simulink model "model1_副本"  (R2023b)
settings: Solver=VariableStepAuto  StartTime=0.0  StopTime=10.0  RelTol=1e-3
undefined symbols (not defined in the file): a558, b523fd510067, DiscIntNeverNeededParam, e0d6, magnitude, Newton, Raphson
libraries: simulink x87, slpidlib x16
(part 1 of 3)
settings Model: Creator=OSCAR4  LastModifiedBy=OSCAR4

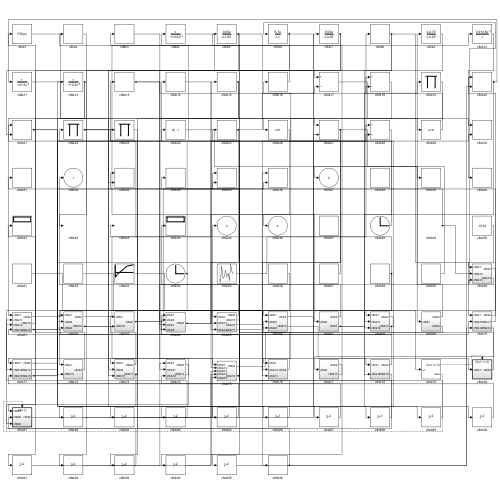
[thumbnail: Simulink's stored preview of the top-level diagram]
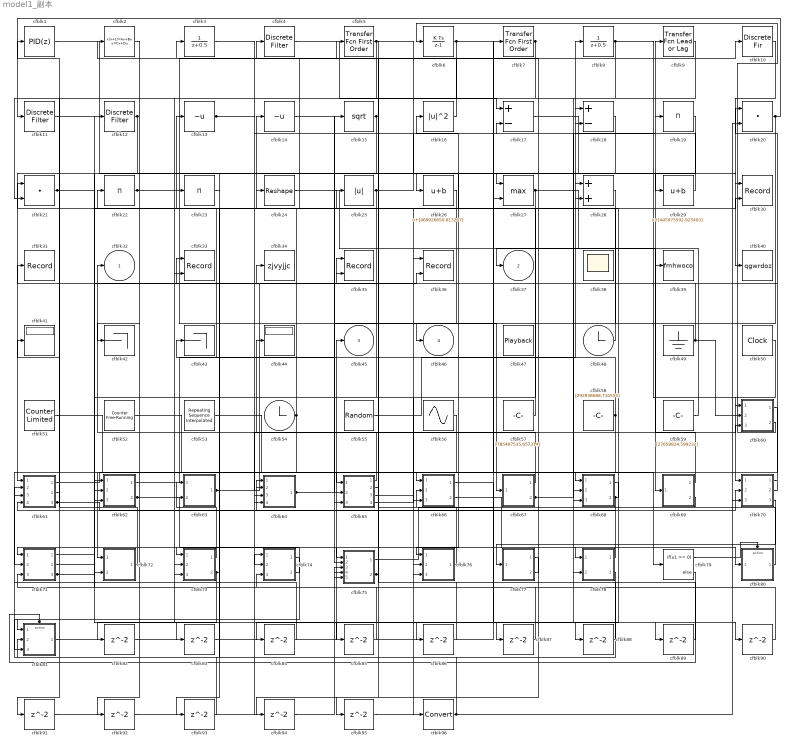
== system model1_副本 ==
  cfblk1 : slpidlib/PID Controller  Controller=PID  Form=Parallel  TimeDomain=Discrete-time  UseExternalTs=off  SampleTime=1  IntegratorMethod=Forward Euler  FilterMethod=Forward Euler  ControllerParametersSource=internal  P=1  I=1  UseKiTs=off  D=0  N=100  UseFilter=on  TunerSelectOption=Transfer Function Based (PID Tuner App)  InitialConditionSource=internal  InitialConditionForIntegrator=0  InitialConditionForFilter=0  DifferentiatorICPrevScaledInput=0  ExternalReset=none  TrackingMode=off  Kt=1  LimitOutput=off  SatLimitsSource=internal  UpperSaturationLimit=inf  LowerSaturationLimit=-inf  LinearizeAsGain=off  AntiWindupMode=none  Kb=1  LimitIntegrator=off  UpperIntegratorSaturationLimit=inf  LowerIntegratorSaturationLimit=-inf  POutMin=[]  POutMax=[]  IOutMin=[]  IOutMax=[]  DOutMin=[]  DOutMax=[]  NOutMin=[]  NOutMax=[]  SumOutMin=[]  SumOutMax=[]  SaturationOutMin=[]  SaturationOutMax=[]  PParamMin=[]  PParamMax=[]  IParamMin=[]  IParamMax=[]  DParamMin=[]  DParamMax=[]  NParamMin=[]  NParamMax=[]  KbParamMin=[]  KbParamMax=[]  KtParamMin=[]  KtParamMax=[]  KbOutMin=[]  KbOutMax=[]  KtOutMin=[]  KtOutMax=[]  IntegratorOutMin=[]  IntegratorOutMax=[]  FilterOutMin=[]  FilterOutMax=[]  SumI1OutMin=[]  SumI1OutMax=[]  SumI2OutMin=[]  SumI2OutMax=[]  SumI3OutMin=[]  SumI3OutMax=[]  SumI4OutMin=[]  SumI4OutMax=[]  SumDOutMin=[]  SumDOutMax=[]  DifferentiatorOutMin=[]  DifferentiatorOutMax=[]  FilterDiffOutCoefMin=[]  FilterDiffOutCoefMax=[]  ReciprocalOutMin=[]  ReciprocalOutMax=[]  SumDenOutMin=[]  SumDenOutMax=[]  SumNumOutMin=[]  SumNumOutMax=[]  DivideOutMin=[]  DivideOutMax=[]  UdiffTsProdOutMin=[]  UdiffTsProdOutMax=[]  NTsProdOutMin=[]  NTsProdOutMax=[]  UintegralTsProdOutMin=[]  UintegralTsProdOutMax=[]  UngainTsProdOutMin=[]  UngainTsProdOutMax=[]  ClampingZeroOutDataTypeStr=Inherit: Inherit via back propagation  ClampingZeroOutMin=[]  ClampingZeroOutMax=[]  FilterDenConstantOutDataTypeStr=Inherit: Inherit via back propagation  FilterDenConstantOutMin=[]  FilterDenConstantOutMax=[]  PCopyOutDataTypeStr=Inherit: Inherit via back propagation  PCopyOutMin=[]  PCopyOutMax=[]  NCopyOutDataTypeStr=Inherit: Inherit via back propagation  NCopyOutMin=[]  NCopyOutMax=[]  IntegratorContinuousStateAttributes=''  IntegratorStateMustResolveToSignalObject=off  IntegratorRTWStateStorageClass=Auto  FilterContinuousStateAttributes=''  FilterStateMustResolveToSignalObject=off  FilterRTWStateStorageClass=Auto  ParallelPVariant=InternalParameters  IdealPVariant=Disabled  IVariant=InternalParameters  DVariant=InternalParameters  IntegratorVariant=Discrete  SatVariant=Disabled  AWVariant=Passthrough  PCopyVariant=Disabled  TRVariant=Disabled  FdbkBlocksVariant=Forward  IdealPFdbkVariant=Disabled  SatFdbkVariant=Disabled  DerivativeFilterVariant=ForwardEulerFilter  NVariant=InternalParameters  NCopyVariant=Disabled  FilterICVariant=InternalICsFilter  IntegratorICVariant=InternalICs  ExternalResetVariant=Disabled  TRSumVariant=Passthrough  SumFdbkVariant=Disabled  SumVariant=Sum_PID  TsampFilterVariant=InternalTs  TsampNgainVariant=Passthrough  TsampIntegralVariant=Disabled_SignalSpec  ExternalSaturationOutDataTypeStr=Inherit: Same as second input
      settings: LibrarySourceBlock=simulink/Discrete/Discrete PID Controller
  cfblk10 : DiscreteFir  SampleTime=1
  cfblk11 : DiscreteFilter  SampleTime=1
  cfblk12 : DiscreteFilter  SampleTime=1
  cfblk13 : UnaryMinus
  cfblk14 : UnaryMinus
  cfblk15 : Sqrt
  cfblk16 : Math  Operator=magnitude^2
  cfblk17 : Sum  Inputs=+-
  cfblk18 : Sum  Inputs=+-
  cfblk19 : Product  Inputs=*
  cfblk2 : DiscreteStateSpace
  cfblk20 : DotProduct  OutDataTypeStr=Inherit: Inherit via internal rule
  cfblk21 : DotProduct  OutDataTypeStr=Inherit: Inherit via internal rule
  cfblk22 : Product  Inputs=*
  cfblk23 : Product  Inputs=*
  cfblk24 : Reshape
  cfblk25 : Abs  SaturateOnIntegerOverflow=off
  cfblk26 : Bias  Bias=[469926650.613267]  SaturateOnIntegerOverflow=off
  cfblk27 : MinMax  Function=max  Inputs=2
  cfblk28 : Sum
  cfblk29 : Bias  Bias=[445975592.923403]  SaturateOnIntegerOverflow=off
  cfblk3 : DiscreteTransferFcn  SampleTime=1
  cfblk30 : Record  FileSettingsInternal="{\"entries\":[{\"content\":{\"excelSettings\":{\"content\":{},\"type\":\"Streamout.ExcelSettings\"}},\"type\":\"Streamout.FileSettingStorage\",\"uuid\":\"\"}],\"packageUris\":[\"http:\\/\\/schema.mathworks.com\\/mf0\\/streamout_blocks\\/R2020a\"],\"version\":\"1.0\"}"  Layout=[1 1]  SignalsInternal="{\"entries\":[{\"content\":{\"signals\":[{\"content\":{\"blockPath\":[],\"dimensions\":[1],\"domain\":\"\",\"lineColor\":\"#a2142f\",\"plots\":[1],\"port\":1,\"sid\":[\"\"],\"signalID\":864,\"signalName\":\"cfblk17\"},\"type\":\"RecordBlkView.Signal\",\"uuid\":\"\"},{\"content\":{\"blockPath\":[],\"dimensions\":[1],\"domain\":\"\",\"lineColor\":\"#139fff\",\"plots\":[1],\"port\":2,\"sid\":[\"\"],\"signalID\":868,\"signalName\":\"cfblk65:3\"},\"type\":\"RecordBlkView.Signal\",\"uuid\":\"\"}]},\"type\":\"RecordBlkView.InputSignals\",\"uuid\":\"\"}],\"packageUris\":[\"http:\\/\\/schema.mathworks.com\\/mf0\\/streamout_blocks\\/R2020a\"],\"version\":\"1.0\"}"  VisualizationBindings="{\"xyplotplugin\":{\"info\":[{\"series\":[{\"bindingParametersList\":[{\"parameter\":\"X-Axis\",\"signalID\":864,\"signalName\":\"cfblk17\"},{\"parameter\":\"Y-Axis\",\"signalID\":868,\"signalName\":\"cfblk65:3\"}],\"seriesID\":27169}],\"subplotID\":1}]}}"  CompatibilityTag=XY
  cfblk31 : Record  FileSettingsInternal="{\"entries\":[{\"content\":{\"excelSettings\":{\"content\":{},\"type\":\"Streamout.ExcelSettings\"}},\"type\":\"Streamout.FileSettingStorage\",\"uuid\":\"\"}],\"packageUris\":[\"http:\\/\\/schema.mathworks.com\\/mf0\\/streamout_blocks\\/R2020a\"],\"version\":\"1.0\"}"  SignalsInternal="{\"entries\":[{\"content\":{\"signals\":[{\"content\":{\"blockPath\":[],\"dimensions\":[1],\"domain\":\"\",\"lineColor\":\"#ff6929\",\"plots\":[1],\"port\":1,\"sid\":[\"\"],\"signalID\":848,\"signalName\":\"cfblk75:2\"},\"type\":\"RecordBlkView.Signal\",\"uuid\":\"\"}]},\"type\":\"RecordBlkView.InputSignals\",\"uuid\":\"\"}],\"packageUris\":[\"http:\\/\\/schema.mathworks.com\\/mf0\\/streamout_blocks\\/R2020a\"],\"version\":\"1.0\"}"  VisualizationBindings="{\"sparklinesplugin\":{\"info\":[{\"bindingParametersList\":[],\"subplotID\":1}]}}"
  cfblk33 : Record  FileSettingsInternal="{\"entries\":[{\"content\":{\"excelSettings\":{\"content\":{},\"type\":\"Streamout.ExcelSettings\"}},\"type\":\"Streamout.FileSettingStorage\",\"uuid\":\"\"}],\"packageUris\":[\"http:\\/\\/schema.mathworks.com\\/mf0\\/streamout_blocks\\/R2020a\"],\"version\":\"1.0\"}"  Layout=[1 1]  SignalsInternal="{\"entries\":[{\"content\":{\"signals\":[{\"content\":{\"blockPath\":[],\"dimensions\":[1],\"domain\":\"\",\"lineColor\":\"#a2142f\",\"plots\":[1],\"port\":1,\"sid\":[\"\"],\"signalID\":872,\"signalName\":\"cfblk75:2\"},\"type\":\"RecordBlkView.Signal\",\"uuid\":\"\"},{\"content\":{\"blockPath\":[],\"dimensions\":[1],\"domain\":\"\",\"lineColor\":\"#139fff\",\"plots\":[1],\"port\":2,\"sid\":[\"\"],\"signalID\":876,\"signalName\":\"cfblk8\"},\"type\":\"RecordBlkView.Signal\",\"uuid\":\"\"}]},\"type\":\"RecordBlkView.InputSignals\",\"uuid\":\"\"}],\"packageUris\":[\"http:\\/\\/schema.mathworks.com\\/mf0\\/streamout_blocks\\/R2020a\"],\"version\":\"1.0\"}"  VisualizationBindings="{\"xyplotplugin\":{\"info\":[{\"series\":[{\"bindingParametersList\":[{\"parameter\":\"X-Axis\",\"signalID\":872,\"signalName\":\"cfblk75:2\"},{\"parameter\":\"Y-Axis\",\"signalID\":876,\"signalName\":\"cfblk8\"}],\"seriesID\":2036}],\"subplotID\":1}]}}"  CompatibilityTag=XY
  cfblk34 : ToWorkspace  VariableName=zjvyjjc  SaveFormat=Timeseries  SampleTime=-1
  cfblk35 : Record  FileSettingsInternal="{\"entries\":[{\"content\":{\"excelSettings\":{\"content\":{},\"type\":\"Streamout.ExcelSettings\"}},\"type\":\"Streamout.FileSettingStorage\",\"uuid\":\"\"}],\"packageUris\":[\"http:\\/\\/schema.mathworks.com\\/mf0\\/streamout_blocks\\/R2020a\"],\"version\":\"1.0\"}"  Layout=[1 1]  SignalsInternal="{\"entries\":[{\"content\":{\"signals\":[{\"content\":{\"blockPath\":[],\"dimensions\":[1],\"domain\":\"\",\"lineColor\":\"#139fff\",\"plots\":[1],\"port\":2,\"sid\":[\"\"],\"signalID\":880,\"signalName\":\"cfblk63\"},\"type\":\"RecordBlkView.Signal\",\"uuid\":\"\"},{\"content\":{\"blockPath\":[],\"dimensions\":[1],\"domain\":\"\",\"lineColor\":\"#a2142f\",\"plots\":[1],\"port\":1,\"sid\":[\"\"],\"signalID\":896,\"signalName\":\"cfblk49\"},\"type\":\"RecordBlkView.Signal\",\"uuid\":\"\"}]},\"type\":\"RecordBlkView.InputSignals\",\"uuid\":\"\"}],\"packageUris\":[\"http:\\/\\/schema.mathworks.com\\/mf0\\/streamout_blocks\\/R2020a\"],\"version\":\"1.0\"}"  VisualizationBindings="{\"xyplotplugin\":{\"info\":[{\"series\":[{\"bindingParametersList\":[{\"parameter\":\"X-Axis\",\"signalID\":896,\"signalName\":\"cfblk49\"},{\"parameter\":\"Y-Axis\",\"signalID\":880,\"signalName\":\"cfblk63\"}],\"seriesID\":60971}],\"subplotID\":1}]}}"  CompatibilityTag=XY
  cfblk36 : Record  FileSettingsInternal="{\"entries\":[{\"content\":{\"excelSettings\":{\"content\":{},\"type\":\"Streamout.ExcelSettings\"}},\"type\":\"Streamout.FileSettingStorage\",\"uuid\":\"\"}],\"packageUris\":[\"http:\\/\\/schema.mathworks.com\\/mf0\\/streamout_blocks\\/R2020a\"],\"version\":\"1.0\"}"  Layout=[1 1]  SignalsInternal="{\"entries\":[{\"content\":{\"signals\":[{\"content\":{\"blockPath\":[],\"dimensions\":[1,1],\"domain\":\"\",\"lineColor\":\"#a2142f\",\"plots\":[1],\"port\":1,\"sid\":[\"\"],\"signalID\":884,\"signalName\":\"cfblk65:4\"},\"type\":\"RecordBlkView.Signal\",\"uuid\":\"\"},{\"content\":{\"blockPath\":[],\"dimensions\":[1,1],\"domain\":\"\",\"lineColor\":\"#139fff\",\"plots\":[1],\"port\":2,\"sid\":[\"\"],\"signalID\":888,\"signalName\":\"cfblk71:3\"},\"type\":\"RecordBlkView.Signal\",\"uuid\":\"\"}]},\"type\":\"RecordBlkView.InputSignals\",\"uuid\":\"\"}],\"packageUris\":[\"http:\\/\\/schema.mathworks.com\\/mf0\\/streamout_blocks\\/R2020a\"],\"version\":\"1.0\"}"  VisualizationBindings="{\"xyplotplugin\":{\"info\":[{\"series\":[{\"bindingParametersList\":[{\"parameter\":\"X-Axis\",\"signalID\":884,\"signalName\":\"cfblk65:4\"},{\"parameter\":\"Y-Axis\",\"signalID\":888,\"signalName\":\"cfblk71:3\"}],\"seriesID\":23987}],\"subplotID\":1}]}}"  CompatibilityTag=XY
  cfblk38 : Scope
      settings: Floating=on
  cfblk39 : ToWorkspace  VariableName=fmhwoco  SaveFormat=Timeseries  SampleTime=-1
  cfblk4 : DiscreteFilter  SampleTime=1
  cfblk40 : ToWorkspace  VariableName=qgwrdoz  SaveFormat=Timeseries  SampleTime=-1
  cfblk41 : Display
  cfblk42 : Terminator
  cfblk43 : Terminator
  cfblk44 : Display
  cfblk47 : Playback  NumPorts=0  PartName=36defed5-e0d6-41a1-a558-b523fd510067
  cfblk48 : Clock
  cfblk49 : Ground
  cfblk5 : simulink/Discrete/Transfer Fcn First Order  PoleZ=0.95  ICPrevOutput=0.0  DoSatur=off
  cfblk50 : DigitalClock
  cfblk51 : simulink/Sources/Counter Limited  uplimit=[223.000000]  tsamp=-1
  cfblk52 : simulink/Sources/Counter Free-Running  NumBits=[22.000000]  tsamp=-1
  cfblk53 : simulink/Sources/Repeating Sequence Interpolated  OutValues=[-505600590.852767, -222429001.362350, 434169832.894922, 629003669.042864, 798997869.181004]  TimeValues=[0 0.1 0.5 0.6 1].'  LookUpMeth=Use Input Nearest  tsamp=0.01  OutMin=[]  OutMax=[]  OutDataTypeStr=double  OutputDataTypeScalingMode=double  OutDataType=fixdt(0,8)  OutScaling=2^-10
  cfblk54 : Clock
  cfblk55 : UniformRandomNumber  Minimum=[-9244758245.197369]  Maximum=[3053319660.851500]  Seed=[9943217.000000]  SampleTime=0.1
  cfblk56 : Sin  Amplitude=[-790585520.472188]  Bias=[947156710.319980]  SampleTime=0
  cfblk57 : Constant  Value=[785497535.657314]  SampleTime=1
  cfblk58 : Constant  Value=[292938688.710555]  SampleTime=1
  cfblk59 : Constant  Value=[27658824.599232]  SampleTime=1
  cfblk6 : DiscreteIntegrator  ICPrevOutput=DiscIntNeverNeededParam  ICPrevScaledInput=DiscIntNeverNeededParam
  cfblk60 : Subsystem
  cfblk61 : Subsystem
  cfblk62 : Subsystem
  cfblk63 : Subsystem
  cfblk64 : Subsystem
  cfblk65 : Subsystem
  cfblk66 : Subsystem
  cfblk67 : Subsystem
  cfblk68 : Subsystem
  cfblk69 : Subsystem
  cfblk7 : simulink/Discrete/Transfer Fcn First Order  PoleZ=0.95  ICPrevOutput=0.0  DoSatur=off
  cfblk70 : Subsystem
  cfblk71 : Subsystem
  cfblk72 : Subsystem
  cfblk73 : Subsystem
  cfblk74 : Subsystem
  cfblk75 : Subsystem
  cfblk76 : Subsystem
  cfblk77 : Subsystem
  cfblk78 : Subsystem
  cfblk79 : If  IfExpression=u1 >= 0  SampleTime=1
  cfblk8 : DiscreteTransferFcn  SampleTime=1
  cfblk80 : Subsystem  TreatAsAtomicUnit=on
  cfblk81 : Subsystem  TreatAsAtomicUnit=on
  cfblk{82..95} (14 alike) : Delay  SampleTime=1
  cfblk9 : simulink/Discrete/Transfer Fcn Lead or Lag  PoleZ=0.95  ZeroZ=0.75  ICPrevOutput=0.0  ICPrevInput=0.0  DoSatur=off
  cfblk96 : DataTypeConversion  SaturateOnIntegerOverflow=off  RndMeth=Floor
  cfblk32 : Outport
  cfblk37 : Outport  Port=2
  cfblk45 : Outport  Port=3
  cfblk46 : Outport  Port=4
  wires:
  cfblk81/1(cfblk2) -> cfblk45/1
  cfblk52/1 -> cfblk96/1
  cfblk1/1 -> cfblk26/1
  cfblk49/1 -> cfblk35/1, cfblk60/2(cfblk12)
  cfblk61/1(cfblk2) -> cfblk65/1(cfblk1)
  cfblk60/1(cfblk2) -> cfblk65/2(cfblk13)
  cfblk54/1 -> cfblk14/1, cfblk64/3(cfblk7)
  cfblk22/1 -> cfblk10/1, cfblk67/1(cfblk1), cfblk90/1
  cfblk62/1(cfblk2) -> cfblk15/1
  cfblk26/1 -> cfblk46/1
  cfblk64/1(cfblk2) -> cfblk66/1(cfblk1), cfblk28/1
  cfblk59/1 -> cfblk37/1
  cfblk16/1 -> cfblk2/1
  cfblk28/1 -> cfblk65/3(cfblk14)
  cfblk63/1(cfblk2) -> cfblk35/2, cfblk60/3(cfblk13)
  cfblk29/1 -> cfblk8/1
  cfblk57/1 -> cfblk4/1
  cfblk69/1(cfblk2) -> cfblk9/1
  cfblk75/1(cfblk2) -> cfblk7/1
  cfblk24/1 -> cfblk69/1(cfblk1)
  cfblk65/1(cfblk2) -> cfblk32/1
  cfblk15/1 -> cfblk61/1(cfblk1), cfblk64/4(cfblk8)
  cfblk60/2(cfblk14) -> cfblk6/1
  cfblk50/1 -> cfblk70/1(cfblk1)
  cfblk51/1 -> cfblk79/1
  cfblk62/2(cfblk10) -> cfblk78/1(cfblk1), cfblk63/2(cfblk16)
  cfblk12/1 -> cfblk81/1(cfblk1), cfblk62/3(cfblk9)
  cfblk69/2(cfblk8) -> cfblk66/2(cfblk8)
  cfblk5/1 -> cfblk29/1, cfblk73/3(cfblk10), cfblk95/1
  cfblk14/1 -> cfblk66/3(cfblk9)
  cfblk48/1 -> cfblk16/1
  cfblk10/1 -> cfblk40/1
  cfblk9/1 -> cfblk78/2(cfblk15)
  cfblk6/1 -> cfblk68/1(cfblk1), cfblk91/1
  cfblk13/1 -> cfblk75/1(cfblk1), cfblk18/2
  cfblk20/1 -> cfblk11/1, cfblk68/2(cfblk11)
  cfblk27/1 -> cfblk75/2(cfblk12), cfblk39/1, cfblk76/3(cfblk11)
  cfblk73/1(cfblk2) -> cfblk63/1(cfblk1)
  cfblk8/1 -> cfblk60/1(cfblk1), cfblk21/2, cfblk33/2
  cfblk56/1 -> cfblk72/1(cfblk1)
  cfblk80/1(cfblk2) -> cfblk22/1
  cfblk76/1(cfblk2) -> cfblk25/1
  cfblk3/1 -> cfblk27/1
  cfblk58/1 -> cfblk13/1, cfblk71/2(cfblk10), cfblk68/3(cfblk12)
  cfblk78/1(cfblk2) -> cfblk64/1(cfblk1)
  cfblk78/2(cfblk16) -> cfblk81/2(cfblk8)
  cfblk70/1(cfblk2) -> cfblk20/1
  cfblk4/1 -> cfblk17/1
  cfblk18/1 -> cfblk73/1(cfblk1)
  cfblk11/1 -> cfblk73/2(cfblk9)
  cfblk74/1(cfblk2) -> cfblk81/3(cfblk9)
  cfblk73/2(cfblk11) -> cfblk23/1, cfblk92/1
  cfblk21/1 -> cfblk86/1, cfblk87/1
  cfblk70/2(cfblk13) -> cfblk34/1
  cfblk17/1 -> cfblk30/1
  cfblk7/1 -> cfblk74/2(cfblk11), cfblk82/1
  cfblk2/1 -> cfblk42/1
  cfblk25/1 -> cfblk17/2, cfblk72/2(cfblk10)
  cfblk70/3(cfblk14) -> cfblk77/1(cfblk1)
  cfblk55/1 -> cfblk18/1
  cfblk74/2(cfblk13) -> cfblk71/1(cfblk1)
  cfblk66/2(cfblk10) -> cfblk80/1(cfblk1)
  cfblk19/1 -> cfblk76/1(cfblk1)
  cfblk71/2(cfblk12) -> cfblk12/1
  cfblk75/2(cfblk16) -> cfblk31/1, cfblk33/1
  cfblk53/1 -> cfblk76/2(cfblk10)
  cfblk67/1(cfblk2) -> cfblk44/1
  cfblk77/2(cfblk17) -> cfblk5/1
  cfblk68/2(cfblk13) -> cfblk21/1, cfblk64/2(cfblk6)
  cfblk65/3(cfblk16) -> cfblk30/2
  cfblk61/2(cfblk14) -> cfblk1/1
  cfblk65/4(cfblk17) -> cfblk36/1
  cfblk71/3(cfblk13) -> cfblk24/1, cfblk36/2
  cfblk72/1(cfblk2) -> cfblk41/1
  cfblk61/3(cfblk15) -> cfblk70/2(cfblk11), cfblk28/2
  cfblk67/2(cfblk7) -> cfblk19/1, cfblk89/1
  cfblk79/1 -> cfblk80/Action
  cfblk79/2 -> cfblk81/Action
  cfblk82/1 -> cfblk27/2
  cfblk71/1(cfblk2) -> cfblk83/1
  cfblk83/1 -> cfblk75/3(cfblk13)
  cfblk65/2(cfblk15) -> cfblk84/1
  cfblk84/1 -> cfblk61/3(cfblk12)
  cfblk68/1(cfblk2) -> cfblk85/1
  cfblk85/1 -> cfblk62/2(cfblk8)
  cfblk86/1 -> cfblk3/1
  cfblk87/1 -> cfblk74/3(cfblk12)
  cfblk66/1(cfblk2) -> cfblk88/1
  cfblk88/1 -> cfblk62/1(cfblk1)
  cfblk89/1 -> cfblk61/4(cfblk13)
  cfblk90/1 -> cfblk71/3(cfblk11)
  cfblk91/1 -> cfblk75/5(cfblk15)
  cfblk92/1 -> cfblk74/1(cfblk1)
  cfblk23/1 -> cfblk93/1
  cfblk93/1 -> cfblk61/2(cfblk11)
  cfblk77/1(cfblk2) -> cfblk94/1
  cfblk94/1 -> cfblk75/4(cfblk14)
  cfblk95/1 -> cfblk70/3(cfblk12)
  cfblk96/1 -> cfblk20/2, cfblk43/1

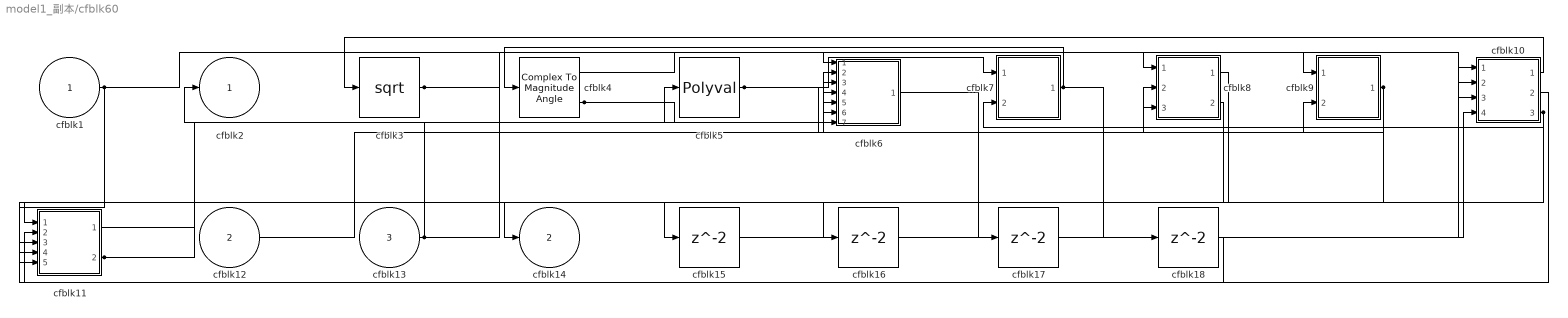
== system model1_副本/cfblk60 ==
  cfblk1 : Inport
  cfblk12 : Inport  Port=2
  cfblk13 : Inport  Port=3
  cfblk10 : Subsystem
  cfblk11 : Subsystem
  cfblk{15..18} (4 alike) : Delay  SampleTime=1
  cfblk3 : Sqrt
  cfblk4 : ComplexToMagnitudeAngle
  cfblk5 : Polyval  Coefs=[ +2.081618890e-019, -1.441693666e-014, +4.719686976e-010, -8.536869453e-006, +1.621573104e-001, -8.087801117e+001 ]
  cfblk6 : Subsystem
  cfblk7 : Subsystem
  cfblk8 : Subsystem
  cfblk9 : Subsystem
  cfblk2 : Outport
  cfblk14 : Outport  Port=2
  wires:
  cfblk5/1 -> cfblk7/1(cfblk1), cfblk9/2(cfblk7)
  cfblk7/1(cfblk2) -> cfblk4/1, cfblk18/1
  cfblk9/1(cfblk2) -> cfblk14/1, cfblk6/6(cfblk16)
  cfblk13/1 -> cfblk2/1, cfblk6/4(cfblk14), cfblk8/3(cfblk15)
  cfblk4/1 -> cfblk6/1(cfblk1)
  cfblk10/1(cfblk2) -> cfblk3/1
  cfblk8/2(cfblk16) -> cfblk11/1(cfblk1)
  cfblk1/1 -> cfblk10/3(cfblk14), cfblk11/3(cfblk9), cfblk9/1(cfblk1)
  cfblk3/1 -> cfblk8/1(cfblk1), cfblk6/5(cfblk15)
  cfblk12/1 -> cfblk8/2(cfblk14)
  cfblk4/2 -> cfblk6/2(cfblk12), cfblk6/7(cfblk17)
  cfblk10/2(cfblk16) -> cfblk11/2(cfblk8)
  cfblk11/2(cfblk12) -> cfblk6/3(cfblk13), cfblk5/1
  cfblk10/3(cfblk17) -> cfblk7/2(cfblk9), cfblk11/5(cfblk11)
  cfblk8/1(cfblk2) -> cfblk15/1
  cfblk15/1 -> cfblk10/1(cfblk1)
  cfblk11/1(cfblk2) -> cfblk16/1
  cfblk16/1 -> cfblk10/4(cfblk15)
  cfblk6/1(cfblk2) -> cfblk17/1
  cfblk17/1 -> cfblk10/2(cfblk13)
  cfblk18/1 -> cfblk11/4(cfblk10)

== system model1_副本/cfblk61 ==
  cfblk1 : Inport
  cfblk11 : Inport  Port=2
  cfblk12 : Inport  Port=3
  cfblk13 : Inport  Port=4
  cfblk10 : Subsystem
  cfblk16 : Delay  SampleTime=1
  cfblk3 : simulink/Discrete/Transfer Fcn First Order  PoleZ=0.95  ICPrevOutput=0.0  DoSatur=off
  cfblk4 : slpidlib/PID Controller (2DOF)  Controller=PID  Form=Parallel  TimeDomain=Discrete-time  UseExternalTs=off  SampleTime=1  IntegratorMethod=Forward Euler  FilterMethod=Forward Euler  ControllerParametersSource=internal  P=1  I=1  UseKiTs=off  D=0  N=100  UseFilter=on  b=1  c=1  TunerSelectOption=Transfer Function Based (PID Tuner App)  InitialConditionSource=internal  InitialConditionForIntegrator=0  InitialConditionForFilter=0  DifferentiatorICPrevScaledInput=0  ExternalReset=none  TrackingMode=off  Kt=1  LimitOutput=off  SatLimitsSource=internal  UpperSaturationLimit=inf  LowerSaturationLimit=-inf  LinearizeAsGain=off  AntiWindupMode=none  Kb=1  LimitIntegrator=off  UpperIntegratorSaturationLimit=inf  LowerIntegratorSaturationLimit=-inf  POutMin=[]  POutMax=[]  IOutMin=[]  IOutMax=[]  DOutMin=[]  DOutMax=[]  NOutMin=[]  NOutMax=[]  bOutMin=[]  bOutMax=[]  cOutMin=[]  cOutMax=[]  SumOutMin=[]  SumOutMax=[]  SaturationOutMin=[]  SaturationOutMax=[]  PParamMin=[]  PParamMax=[]  IParamMin=[]  IParamMax=[]  DParamMin=[]  DParamMax=[]  NParamMin=[]  NParamMax=[]  bParamMin=[]  bParamMax=[]  cParamMin=[]  cParamMax=[]  KbParamMin=[]  KbParamMax=[]  KtParamMin=[]  KtParamMax=[]  KbOutMin=[]  KbOutMax=[]  KtOutMin=[]  KtOutMax=[]  IntegratorOutMin=[]  IntegratorOutMax=[]  FilterOutMin=[]  FilterOutMax=[]  SumI1OutMin=[]  SumI1OutMax=[]  SumI2OutMin=[]  SumI2OutMax=[]  SumI3OutMin=[]  SumI3OutMax=[]  SumI4OutMin=[]  SumI4OutMax=[]  SumDOutMin=[]  SumDOutMax=[]  Sum1OutMin=[]  Sum1OutMax=[]  Sum2OutMin=[]  Sum2OutMax=[]  Sum3OutMin=[]  Sum3OutMax=[]  DifferentiatorOutMin=[]  DifferentiatorOutMax=[]  FilterDiffOutCoefMin=[]  FilterDiffOutCoefMax=[]  ReciprocalOutMin=[]  ReciprocalOutMax=[]  SumDenOutMin=[]  SumDenOutMax=[]  SumNumOutMin=[]  SumNumOutMax=[]  DivideOutMin=[]  DivideOutMax=[]  UdiffTsProdOutMin=[]  UdiffTsProdOutMax=[]  NTsProdOutMin=[]  NTsProdOutMax=[]  UintegralTsProdOutMin=[]  UintegralTsProdOutMax=[]  UngainTsProdOutMin=[]  UngainTsProdOutMax=[]  ClampingZeroOutDataTypeStr=Inherit: Inherit via back propagation  ClampingZeroOutMin=[]  ClampingZeroOutMax=[]  FilterDenConstantOutDataTypeStr=Inherit: Inherit via back propagation  FilterDenConstantOutMin=[]  FilterDenConstantOutMax=[]  PCopyOutDataTypeStr=Inherit: Inherit via back propagation  PCopyOutMin=[]  PCopyOutMax=[]  NCopyOutDataTypeStr=Inherit: Inherit via back propagation  NCopyOutMin=[]  NCopyOutMax=[]  IntegratorContinuousStateAttributes=''  IntegratorStateMustResolveToSignalObject=off  IntegratorRTWStateStorageClass=Auto  FilterContinuousStateAttributes=''  FilterStateMustResolveToSignalObject=off  FilterRTWStateStorageClass=Auto  ParallelPVariant=InternalParameters  IdealPVariant=Disabled  IVariant=InternalParameters  DVariant=InternalParameters  bVariant=InternalParameters  cVariant=InternalParameters  IntegratorVariant=Discrete  SatVariant=Disabled  AWVariant=Passthrough  PCopyVariant=Disabled  TRVariant=Disabled  FdbkBlocksVariant=Forward  IdealPFdbkVariant=Disabled  SatFdbkVariant=Disabled  DerivativeFilterVariant=ForwardEulerFilter  NVariant=InternalParameters  NCopyVariant=Disabled  FilterICVariant=InternalICsFilter  IntegratorICVariant=InternalICs  ExternalResetVariant=Disabled  TRSumVariant=Passthrough  SumFdbkVariant=Disabled  SumVariant=Sum_PID  TsampFilterVariant=InternalTs  TsampNgainVariant=Passthrough  TsampIntegralVariant=Disabled_SignalSpec  ExternalSaturationOutDataTypeStr=Inherit: Same as second input
      settings: LibrarySourceBlock=simulink/Discrete/Discrete PID Controller (2DOF)
  cfblk5 : Sum  Inputs=+
  cfblk6 : simulink/Math Operations/MinMax Running Resettable  Function=min  vinit=0.0
  cfblk7 : Constant  Value=[70606175.934599]  SampleTime=1
  cfblk8 : Subsystem
  cfblk9 : Subsystem
  cfblk2 : Outport
  cfblk14 : Outport  Port=2
  cfblk15 : Outport  Port=3
  wires:
  cfblk13/1 -> cfblk15/1
  cfblk9/1(cfblk2) -> cfblk5/1, cfblk6/2
  cfblk10/1(cfblk2) -> cfblk4/1
  cfblk11/1 -> cfblk3/1
  cfblk3/1 -> cfblk8/1(cfblk1)
  cfblk1/1 -> cfblk2/1
  cfblk7/1 -> cfblk10/1(cfblk1)
  cfblk4/1 -> cfblk9/1(cfblk1)
  cfblk8/1(cfblk2) -> cfblk10/2(cfblk11)
  cfblk6/1 -> cfblk14/1
  cfblk12/1 -> cfblk4/2
  cfblk8/2(cfblk11) -> cfblk9/2(cfblk14)
  cfblk8/3(cfblk12) -> cfblk9/3(cfblk15)
  cfblk8/4(cfblk13) -> cfblk6/1
  cfblk5/1 -> cfblk16/1
  cfblk16/1 -> cfblk10/3(cfblk12)

== system model1_副本/cfblk62 ==
  cfblk1 : Inport
  cfblk8 : Inport  Port=2
  cfblk9 : Inport  Port=3
  cfblk11 : Delay  SampleTime=1
  cfblk12 : Delay  SampleTime=1
  cfblk3 : DiscreteFilter  SampleTime=1
  cfblk4 : Delay  DelayLengthSource=Input port  SampleTime=1
      settings: InputPortMap=u0,p1
  cfblk5 : MinMax  Inputs=3
  cfblk6 : Constant  Value=[551112500.517372]  SampleTime=1
  cfblk7 : Subsystem
  cfblk2 : Outport
  cfblk10 : Outport  Port=2
  wires:
  cfblk6/1 -> cfblk3/1, cfblk7/3(cfblk8)
  cfblk3/1 -> cfblk5/1
  cfblk8/1 -> cfblk4/1, cfblk7/1(cfblk1)
  cfblk4/1 -> cfblk7/2(cfblk7), cfblk11/1
  cfblk5/1 -> cfblk4/2
  cfblk1/1 -> cfblk2/1
  cfblk9/1 -> cfblk10/1, cfblk7/4(cfblk9)
  cfblk11/1 -> cfblk5/2
  cfblk7/1(cfblk2) -> cfblk12/1
  cfblk12/1 -> cfblk5/3

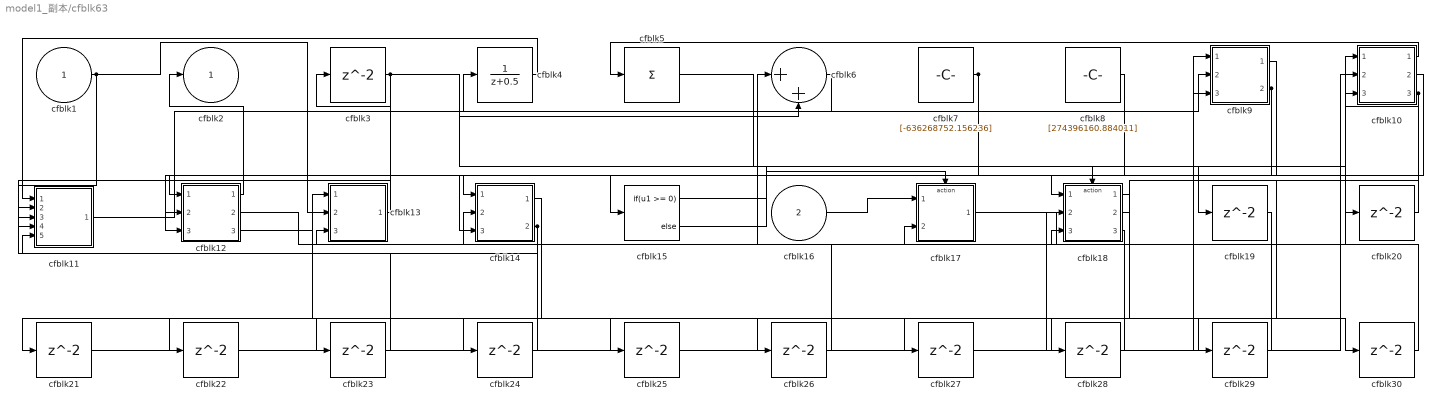
== system model1_副本/cfblk63 ==
  cfblk1 : Inport
  cfblk16 : Inport  Port=2
  cfblk10 : Subsystem
  cfblk11 : Subsystem
  cfblk12 : Subsystem
  cfblk13 : Subsystem
  cfblk14 : Subsystem
  cfblk15 : If  IfExpression=u1 >= 0  SampleTime=1
  cfblk17 : Subsystem  TreatAsAtomicUnit=on
  cfblk18 : Subsystem  TreatAsAtomicUnit=on
  cfblk{3,19..30} (13 alike) : Delay  SampleTime=1
  cfblk4 : DiscreteTransferFcn  SampleTime=1
  cfblk5 : Sum  Inputs=+
  cfblk6 : Sum  Inputs=|++
  cfblk7 : Constant  Value=[-636268752.156236]  SampleTime=1
  cfblk8 : Constant  Value=[274396160.884011]  SampleTime=1
  cfblk9 : Subsystem
  cfblk2 : Outport
  wires:
  cfblk12/1(cfblk2) -> cfblk2/1
  cfblk7/1 -> cfblk14/1(cfblk1), cfblk12/2(cfblk5)
  cfblk16/1 -> cfblk17/1(cfblk1)
  cfblk17/1(cfblk2) -> cfblk10/1(cfblk1)
  cfblk8/1 -> cfblk18/1(cfblk1)
  cfblk1/1 -> cfblk13/2(cfblk14), cfblk11/2(cfblk9)
  cfblk10/1(cfblk2) -> cfblk5/1
  cfblk6/1 -> cfblk4/1
  cfblk11/1(cfblk2) -> cfblk9/2(cfblk6)
  cfblk4/1 -> cfblk11/1(cfblk1)
  cfblk13/1(cfblk2) -> cfblk3/1
  cfblk3/1 -> cfblk6/2, cfblk11/4(cfblk11), cfblk19/1
  cfblk12/2(cfblk7) -> cfblk14/2(cfblk14)
  cfblk9/1(cfblk2) -> cfblk15/1
  cfblk9/2(cfblk8) -> cfblk12/1(cfblk1), cfblk12/3(cfblk6)
  cfblk14/2(cfblk16) -> cfblk22/1, cfblk23/1, cfblk24/1
  cfblk10/2(cfblk10) -> cfblk14/3(cfblk15)
  cfblk10/3(cfblk11) -> cfblk25/1, cfblk29/1
  cfblk15/1 -> cfblk17/Action
  cfblk15/2 -> cfblk18/Action
  cfblk19/1 -> cfblk13/3(cfblk15)
  cfblk5/1 -> cfblk20/1
  cfblk20/1 -> cfblk10/3(cfblk9)
  cfblk14/1(cfblk2) -> cfblk21/1
  cfblk21/1 -> cfblk10/2(cfblk8)
  cfblk22/1 -> cfblk9/3(cfblk7)
  cfblk23/1 -> cfblk11/3(cfblk10)
  cfblk24/1 -> cfblk11/5(cfblk12)
  cfblk25/1 -> cfblk18/2(cfblk6)
  cfblk18/1(cfblk2) -> cfblk26/1
  cfblk26/1 -> cfblk13/1(cfblk1)
  cfblk18/2(cfblk8) -> cfblk27/1
  cfblk27/1 -> cfblk9/1(cfblk1)
  cfblk18/3(cfblk9) -> cfblk28/1
  cfblk28/1 -> cfblk17/2(cfblk8)
  cfblk29/1 -> cfblk18/3(cfblk7)
  cfblk12/3(cfblk8) -> cfblk30/1
  cfblk30/1 -> cfblk6/1

== system model1_副本/cfblk64 ==
  cfblk1 : Inport
  cfblk6 : Inport  Port=2
  cfblk7 : Inport  Port=3
  cfblk8 : Inport  Port=4
  cfblk3 : Delay  DelayLengthSource=Input port  SampleTime=1
      settings: InputPortMap=u0,p1
  cfblk4 : MinMax
  cfblk5 : Constant  Value=[-395344255.806341]  SampleTime=1
  cfblk2 : Outport
  wires:
  cfblk6/1 -> cfblk4/1
  cfblk1/1 -> cfblk3/1
  cfblk5/1 -> cfblk3/2
  cfblk7/1 -> cfblk2/1

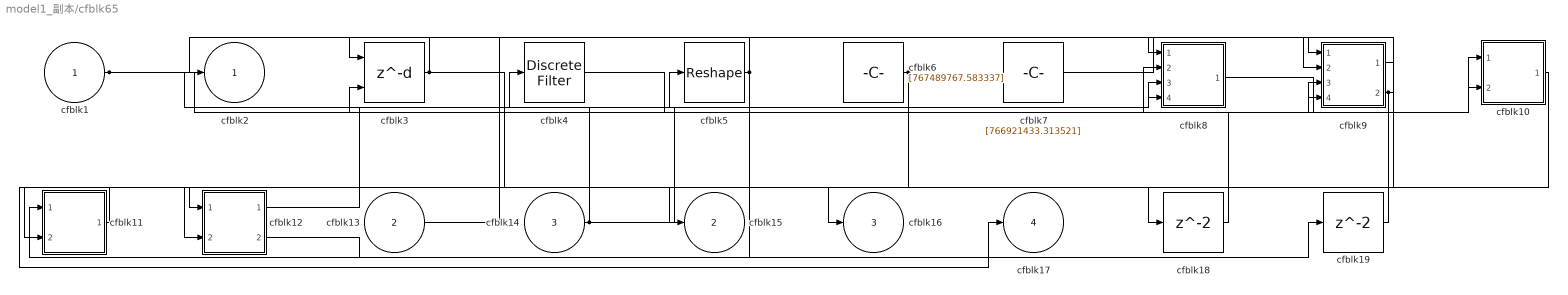
== system model1_副本/cfblk65 ==
  cfblk1 : Inport
  cfblk13 : Inport  Port=2
  cfblk14 : Inport  Port=3
  cfblk10 : Subsystem
  cfblk11 : Subsystem
  cfblk12 : Subsystem
  cfblk18 : Delay  SampleTime=1
  cfblk19 : Delay  SampleTime=1
  cfblk3 : Delay  DelayLengthSource=Input port  SampleTime=1
      settings: InputPortMap=u0,p1
  cfblk4 : DiscreteFilter  SampleTime=1
  cfblk5 : Reshape
  cfblk6 : Constant  Value=[767489767.583337]  SampleTime=1
  cfblk7 : Constant  Value=[766921433.313521]  SampleTime=1
  cfblk8 : Subsystem
  cfblk9 : Subsystem
  cfblk2 : Outport
  cfblk15 : Outport  Port=2
  cfblk16 : Outport  Port=3
  cfblk17 : Outport  Port=4
  wires:
  cfblk14/1 -> cfblk4/1, cfblk8/3(cfblk10)
  cfblk13/1 -> cfblk9/1(cfblk1)
  cfblk5/1 -> cfblk11/1(cfblk1), cfblk3/1
  cfblk11/1(cfblk2) -> cfblk17/1
  cfblk8/1(cfblk2) -> cfblk10/1(cfblk1)
  cfblk12/1(cfblk2) -> cfblk5/1
  cfblk9/1(cfblk2) -> cfblk11/2(cfblk9)
  cfblk7/1 -> cfblk9/2(cfblk14)
  cfblk4/1 -> cfblk10/2(cfblk7)
  cfblk6/1 -> cfblk12/1(cfblk1), cfblk15/1
  cfblk1/1 -> cfblk9/3(cfblk15), cfblk8/4(cfblk11)
  cfblk9/2(cfblk17) -> cfblk8/1(cfblk1), cfblk3/2
  cfblk10/1(cfblk2) -> cfblk12/2(cfblk7)
  cfblk3/1 -> cfblk16/1, cfblk2/1, cfblk18/1
  cfblk18/1 -> cfblk8/2(cfblk9)
  cfblk12/2(cfblk8) -> cfblk19/1
  cfblk19/1 -> cfblk9/4(cfblk16)

== system model1_副本/cfblk66 ==
  cfblk1 : Inport
  cfblk8 : Inport  Port=2
  cfblk9 : Inport  Port=3
  cfblk3 : DiscreteZeroPole  Poles=[0 0.5]  Gain=1
  cfblk4 : simulink/Discrete/Transfer Fcn Real Zero  ZeroZ=0.75  ICPrevInput=0.0  DoSatur=off
  cfblk5 : Math  Operator=hermitian
  cfblk6 : Constant  Value=[794654116.084426]  SampleTime=1
  cfblk7 : Constant  Value=[-838477001.081016]  SampleTime=1
  cfblk2 : Outport
  cfblk10 : Outport  Port=2
  wires:
  cfblk1/1 -> cfblk4/1
  cfblk6/1 -> cfblk3/1
  cfblk5/1 -> cfblk2/1
  cfblk8/1 -> cfblk5/1
  cfblk3/1 -> cfblk10/1

== system model1_副本/cfblk67 ==
  cfblk1 : Inport
  cfblk{10..14} (5 alike) : Delay  SampleTime=1
  cfblk3 : slpidlib/PID Controller (2DOF)  Controller=PID  Form=Parallel  TimeDomain=Discrete-time  UseExternalTs=off  SampleTime=1  IntegratorMethod=Forward Euler  FilterMethod=Forward Euler  ControllerParametersSource=internal  P=1  I=1  UseKiTs=off  D=0  N=100  UseFilter=on  b=1  c=1  TunerSelectOption=Transfer Function Based (PID Tuner App)  InitialConditionSource=internal  InitialConditionForIntegrator=0  InitialConditionForFilter=0  DifferentiatorICPrevScaledInput=0  ExternalReset=none  TrackingMode=off  Kt=1  LimitOutput=off  SatLimitsSource=internal  UpperSaturationLimit=inf  LowerSaturationLimit=-inf  LinearizeAsGain=off  AntiWindupMode=none  Kb=1  LimitIntegrator=off  UpperIntegratorSaturationLimit=inf  LowerIntegratorSaturationLimit=-inf  POutMin=[]  POutMax=[]  IOutMin=[]  IOutMax=[]  DOutMin=[]  DOutMax=[]  NOutMin=[]  NOutMax=[]  bOutMin=[]  bOutMax=[]  cOutMin=[]  cOutMax=[]  SumOutMin=[]  SumOutMax=[]  SaturationOutMin=[]  SaturationOutMax=[]  PParamMin=[]  PParamMax=[]  IParamMin=[]  IParamMax=[]  DParamMin=[]  DParamMax=[]  NParamMin=[]  NParamMax=[]  bParamMin=[]  bParamMax=[]  cParamMin=[]  cParamMax=[]  KbParamMin=[]  KbParamMax=[]  KtParamMin=[]  KtParamMax=[]  KbOutMin=[]  KbOutMax=[]  KtOutMin=[]  KtOutMax=[]  IntegratorOutMin=[]  IntegratorOutMax=[]  FilterOutMin=[]  FilterOutMax=[]  SumI1OutMin=[]  SumI1OutMax=[]  SumI2OutMin=[]  SumI2OutMax=[]  SumI3OutMin=[]  SumI3OutMax=[]  SumI4OutMin=[]  SumI4OutMax=[]  SumDOutMin=[]  SumDOutMax=[]  Sum1OutMin=[]  Sum1OutMax=[]  Sum2OutMin=[]  Sum2OutMax=[]  Sum3OutMin=[]  Sum3OutMax=[]  DifferentiatorOutMin=[]  DifferentiatorOutMax=[]  FilterDiffOutCoefMin=[]  FilterDiffOutCoefMax=[]  ReciprocalOutMin=[]  ReciprocalOutMax=[]  SumDenOutMin=[]  SumDenOutMax=[]  SumNumOutMin=[]  SumNumOutMax=[]  DivideOutMin=[]  DivideOutMax=[]  UdiffTsProdOutMin=[]  UdiffTsProdOutMax=[]  NTsProdOutMin=[]  NTsProdOutMax=[]  UintegralTsProdOutMin=[]  UintegralTsProdOutMax=[]  UngainTsProdOutMin=[]  UngainTsProdOutMax=[]  ClampingZeroOutDataTypeStr=Inherit: Inherit via back propagation  ClampingZeroOutMin=[]  ClampingZeroOutMax=[]  FilterDenConstantOutDataTypeStr=Inherit: Inherit via back propagation  FilterDenConstantOutMin=[]  FilterDenConstantOutMax=[]  PCopyOutDataTypeStr=Inherit: Inherit via back propagation  PCopyOutMin=[]  PCopyOutMax=[]  NCopyOutDataTypeStr=Inherit: Inherit via back propagation  NCopyOutMin=[]  NCopyOutMax=[]  IntegratorContinuousStateAttributes=''  IntegratorStateMustResolveToSignalObject=off  IntegratorRTWStateStorageClass=Auto  FilterContinuousStateAttributes=''  FilterStateMustResolveToSignalObject=off  FilterRTWStateStorageClass=Auto  ParallelPVariant=InternalParameters  IdealPVariant=Disabled  IVariant=InternalParameters  DVariant=InternalParameters  bVariant=InternalParameters  cVariant=InternalParameters  IntegratorVariant=Discrete  SatVariant=Disabled  AWVariant=Passthrough  PCopyVariant=Disabled  TRVariant=Disabled  FdbkBlocksVariant=Forward  IdealPFdbkVariant=Disabled  SatFdbkVariant=Disabled  DerivativeFilterVariant=ForwardEulerFilter  NVariant=InternalParameters  NCopyVariant=Disabled  FilterICVariant=InternalICsFilter  IntegratorICVariant=InternalICs  ExternalResetVariant=Disabled  TRSumVariant=Passthrough  SumFdbkVariant=Disabled  SumVariant=Sum_PID  TsampFilterVariant=InternalTs  TsampNgainVariant=Passthrough  TsampIntegralVariant=Disabled_SignalSpec  ExternalSaturationOutDataTypeStr=Inherit: Same as second input
      settings: LibrarySourceBlock=simulink/Discrete/Discrete PID Controller (2DOF)
  cfblk4 : PermuteDimensions
  cfblk5 : MinMax  Inputs=2
  cfblk6 : If  IfExpression=u1 >= 0  SampleTime=1
  cfblk8 : Subsystem  TreatAsAtomicUnit=on
  cfblk9 : Subsystem  TreatAsAtomicUnit=on
  cfblk2 : Outport
  cfblk7 : Outport  Port=2
  wires:
  cfblk8/1(cfblk2) -> cfblk2/1
  cfblk9/1(cfblk2) -> cfblk4/1
  cfblk5/1 -> cfblk8/2(cfblk12)
  cfblk1/1 -> cfblk5/1, cfblk8/4(cfblk14)
  cfblk8/3(cfblk16) -> cfblk7/1
  cfblk4/1 -> cfblk3/2, cfblk11/1
  cfblk9/3(cfblk16) -> cfblk3/1, cfblk14/1
  cfblk6/1 -> cfblk8/Action
  cfblk6/2 -> cfblk9/Action
  cfblk8/2(cfblk15) -> cfblk10/1
  cfblk10/1 -> cfblk6/1
  cfblk11/1 -> cfblk9/1(cfblk1)
  cfblk3/1 -> cfblk12/1
  cfblk12/1 -> cfblk8/1(cfblk1)
  cfblk9/2(cfblk15) -> cfblk13/1
  cfblk13/1 -> cfblk8/3(cfblk13)
  cfblk14/1 -> cfblk5/2

== system model1_副本/cfblk68 ==
  cfblk1 : Inport
  cfblk11 : Inport  Port=2
  cfblk12 : Inport  Port=3
  cfblk10 : Subsystem
  cfblk14 : Delay  SampleTime=1
  cfblk15 : Delay  SampleTime=1
  cfblk3 : slpidlib/PID Controller (2DOF)  Controller=PID  Form=Parallel  TimeDomain=Discrete-time  UseExternalTs=off  SampleTime=1  IntegratorMethod=Forward Euler  FilterMethod=Forward Euler  ControllerParametersSource=internal  P=1  I=1  UseKiTs=off  D=0  N=100  UseFilter=on  b=1  c=1  TunerSelectOption=Transfer Function Based (PID Tuner App)  InitialConditionSource=internal  InitialConditionForIntegrator=0  InitialConditionForFilter=0  DifferentiatorICPrevScaledInput=0  ExternalReset=none  TrackingMode=off  Kt=1  LimitOutput=off  SatLimitsSource=internal  UpperSaturationLimit=inf  LowerSaturationLimit=-inf  LinearizeAsGain=off  AntiWindupMode=none  Kb=1  LimitIntegrator=off  UpperIntegratorSaturationLimit=inf  LowerIntegratorSaturationLimit=-inf  POutMin=[]  POutMax=[]  IOutMin=[]  IOutMax=[]  DOutMin=[]  DOutMax=[]  NOutMin=[]  NOutMax=[]  bOutMin=[]  bOutMax=[]  cOutMin=[]  cOutMax=[]  SumOutMin=[]  SumOutMax=[]  SaturationOutMin=[]  SaturationOutMax=[]  PParamMin=[]  PParamMax=[]  IParamMin=[]  IParamMax=[]  DParamMin=[]  DParamMax=[]  NParamMin=[]  NParamMax=[]  bParamMin=[]  bParamMax=[]  cParamMin=[]  cParamMax=[]  KbParamMin=[]  KbParamMax=[]  KtParamMin=[]  KtParamMax=[]  KbOutMin=[]  KbOutMax=[]  KtOutMin=[]  KtOutMax=[]  IntegratorOutMin=[]  IntegratorOutMax=[]  FilterOutMin=[]  FilterOutMax=[]  SumI1OutMin=[]  SumI1OutMax=[]  SumI2OutMin=[]  SumI2OutMax=[]  SumI3OutMin=[]  SumI3OutMax=[]  SumI4OutMin=[]  SumI4OutMax=[]  SumDOutMin=[]  SumDOutMax=[]  Sum1OutMin=[]  Sum1OutMax=[]  Sum2OutMin=[]  Sum2OutMax=[]  Sum3OutMin=[]  Sum3OutMax=[]  DifferentiatorOutMin=[]  DifferentiatorOutMax=[]  FilterDiffOutCoefMin=[]  FilterDiffOutCoefMax=[]  ReciprocalOutMin=[]  ReciprocalOutMax=[]  SumDenOutMin=[]  SumDenOutMax=[]  SumNumOutMin=[]  SumNumOutMax=[]  DivideOutMin=[]  DivideOutMax=[]  UdiffTsProdOutMin=[]  UdiffTsProdOutMax=[]  NTsProdOutMin=[]  NTsProdOutMax=[]  UintegralTsProdOutMin=[]  UintegralTsProdOutMax=[]  UngainTsProdOutMin=[]  UngainTsProdOutMax=[]  ClampingZeroOutDataTypeStr=Inherit: Inherit via back propagation  ClampingZeroOutMin=[]  ClampingZeroOutMax=[]  FilterDenConstantOutDataTypeStr=Inherit: Inherit via back propagation  FilterDenConstantOutMin=[]  FilterDenConstantOutMax=[]  PCopyOutDataTypeStr=Inherit: Inherit via back propagation  PCopyOutMin=[]  PCopyOutMax=[]  NCopyOutDataTypeStr=Inherit: Inherit via back propagation  NCopyOutMin=[]  NCopyOutMax=[]  IntegratorContinuousStateAttributes=''  IntegratorStateMustResolveToSignalObject=off  IntegratorRTWStateStorageClass=Auto  FilterContinuousStateAttributes=''  FilterStateMustResolveToSignalObject=off  FilterRTWStateStorageClass=Auto  ParallelPVariant=InternalParameters  IdealPVariant=Disabled  IVariant=InternalParameters  DVariant=InternalParameters  bVariant=InternalParameters  cVariant=InternalParameters  IntegratorVariant=Discrete  SatVariant=Disabled  AWVariant=Passthrough  PCopyVariant=Disabled  TRVariant=Disabled  FdbkBlocksVariant=Forward  IdealPFdbkVariant=Disabled  SatFdbkVariant=Disabled  DerivativeFilterVariant=ForwardEulerFilter  NVariant=InternalParameters  NCopyVariant=Disabled  FilterICVariant=InternalICsFilter  IntegratorICVariant=InternalICs  ExternalResetVariant=Disabled  TRSumVariant=Passthrough  SumFdbkVariant=Disabled  SumVariant=Sum_PID  TsampFilterVariant=InternalTs  TsampNgainVariant=Passthrough  TsampIntegralVariant=Disabled_SignalSpec  ExternalSaturationOutDataTypeStr=Inherit: Same as second input
      settings: LibrarySourceBlock=simulink/Discrete/Discrete PID Controller (2DOF)
  cfblk4 : Sum  Inputs=|++
  cfblk5 : UnaryMinus
  cfblk6 : Sum  Inputs=+
  cfblk7 : Reshape
  cfblk8 : Subsystem
  cfblk9 : Subsystem
  cfblk2 : Outport
  cfblk13 : Outport  Port=2
  wires:
  cfblk12/1 -> cfblk4/1
  cfblk8/1(cfblk2) -> cfblk4/2
  cfblk9/1(cfblk2) -> cfblk8/1(cfblk1)
  cfblk4/1 -> cfblk5/1
  cfblk5/1 -> cfblk6/1
  cfblk7/1 -> cfblk13/1
  cfblk10/1(cfblk2) -> cfblk3/2, cfblk9/3(cfblk10)
  cfblk8/2(cfblk8) -> cfblk7/1
  cfblk11/1 -> cfblk2/1
  cfblk3/1 -> cfblk9/2(cfblk9)
  cfblk1/1 -> cfblk10/1(cfblk1)
  cfblk6/1 -> cfblk14/1
  cfblk14/1 -> cfblk3/1
  cfblk8/3(cfblk9) -> cfblk15/1
  cfblk15/1 -> cfblk9/1(cfblk1)

== system model1_副本/cfblk69 ==
  cfblk1 : Inport
  cfblk{9..12} (4 alike) : Delay  SampleTime=1
  cfblk3 : Trigonometry
  cfblk4 : Subsystem
  cfblk5 : Subsystem
  cfblk6 : Subsystem
  cfblk7 : Subsystem
  cfblk2 : Outport
  cfblk8 : Outport  Port=2
  wires:
  cfblk4/1(cfblk2) -> cfblk5/1(cfblk1), cfblk5/4(cfblk15), cfblk7/1(cfblk1)
  cfblk3/1 -> cfblk2/1, cfblk12/1
  cfblk1/1 -> cfblk4/1(cfblk1)
  cfblk7/1(cfblk2) -> cfblk5/2(cfblk13), cfblk6/2(cfblk8), cfblk8/1
  cfblk6/1(cfblk2) -> cfblk3/1, cfblk11/1
  cfblk5/2(cfblk16) -> cfblk6/3(cfblk9), cfblk10/1
  cfblk5/1(cfblk2) -> cfblk9/1
  cfblk9/1 -> cfblk4/2(cfblk7)
  cfblk10/1 -> cfblk4/3(cfblk8)
  cfblk11/1 -> cfblk5/3(cfblk14)
  cfblk12/1 -> cfblk6/1(cfblk1)

== system model1_副本/cfblk70 ==
  cfblk1 : Inport
  cfblk11 : Inport  Port=2
  cfblk12 : Inport  Port=3
  cfblk10 : Subsystem
  cfblk15 : Delay  SampleTime=1
  cfblk3 : Delay  SampleTime=1
  cfblk4 : ComplexToMagnitudeAngle
  cfblk5 : Constant  Value=[669947679.945022]  SampleTime=1
  cfblk6 : Constant  Value=[216710938.068503]  SampleTime=1
  cfblk7 : Constant  Value=[-742604849.237621]  SampleTime=1
  cfblk8 : Constant  Value=[-888816858.578035]  SampleTime=1
  cfblk9 : Constant  Value=[120983983.707112]  SampleTime=1
  cfblk2 : Outport
  cfblk13 : Outport  Port=2
  cfblk14 : Outport  Port=3
  wires:
  cfblk6/1 -> cfblk4/1
  cfblk3/1 -> cfblk10/1(cfblk1)
  cfblk5/1 -> cfblk14/1
  cfblk1/1 -> cfblk2/1
  cfblk4/1 -> cfblk10/2(cfblk9)
  cfblk7/1 -> cfblk10/3(cfblk10)
  cfblk9/1 -> cfblk13/1
  cfblk10/1(cfblk2) -> cfblk15/1
  cfblk15/1 -> cfblk3/1

== system model1_副本/cfblk71 ==
  cfblk1 : Inport
  cfblk10 : Inport  Port=2
  cfblk11 : Inport  Port=3
  cfblk14 : Delay  SampleTime=1
  cfblk15 : Delay  SampleTime=1
  cfblk3 : DiscreteZeroPole  Poles=[0 0.5]  Gain=1
  cfblk4 : DiscreteFir  SampleTime=1
  cfblk5 : simulink/Math Operations/MinMax Running Resettable  Function=min  vinit=0.0
  cfblk6 : MinMax  Function=max  Inputs=3
  cfblk7 : Constant  Value=[-821568701.362918]  SampleTime=1
  cfblk8 : Subsystem
  cfblk9 : Subsystem
  cfblk2 : Outport
  cfblk12 : Outport  Port=2
  cfblk13 : Outport  Port=3
  wires:
  cfblk10/1 -> cfblk8/1(cfblk1)
  cfblk1/1 -> cfblk12/1, cfblk8/4(cfblk13)
  cfblk11/1 -> cfblk9/1(cfblk1)
  cfblk7/1 -> cfblk2/1, cfblk5/2
  cfblk5/1 -> cfblk6/1
  cfblk4/1 -> cfblk3/1
  cfblk6/1 -> cfblk13/1
  cfblk8/1(cfblk2) -> cfblk9/2(cfblk12)
  cfblk8/2(cfblk14) -> cfblk4/1
  cfblk8/3(cfblk15) -> cfblk6/2
  cfblk9/2(cfblk14) -> cfblk5/1
  cfblk8/4(cfblk16) -> cfblk9/3(cfblk13)
  cfblk9/3(cfblk15) -> cfblk6/3
  cfblk9/1(cfblk2) -> cfblk14/1
  cfblk14/1 -> cfblk8/3(cfblk12)
  cfblk3/1 -> cfblk15/1
  cfblk15/1 -> cfblk8/2(cfblk11)

== system model1_副本/cfblk72 ==
  cfblk1 : Inport
  cfblk10 : Inport  Port=2
  cfblk{11..16} (6 alike) : Delay  SampleTime=1
  cfblk3 : UnitDelay  HasFrameUpgradeWarning=on
  cfblk4 : Sum
  cfblk5 : Subsystem
  cfblk6 : Subsystem
  cfblk7 : Subsystem
  cfblk8 : Subsystem
  cfblk9 : Subsystem
  cfblk2 : Outport
  wires:
  cfblk1/1 -> cfblk3/1
  cfblk3/1 -> cfblk5/1(cfblk1), cfblk4/2, cfblk5/2(cfblk9)
  cfblk7/1(cfblk2) -> cfblk6/1(cfblk1)
  cfblk4/1 -> cfblk2/1
  cfblk10/1 -> cfblk7/1(cfblk1), cfblk5/3(cfblk10)
  cfblk5/1(cfblk2) -> cfblk8/1(cfblk1), cfblk8/3(cfblk11)
  cfblk8/1(cfblk2) -> cfblk7/2(cfblk4)
  cfblk6/1(cfblk2) -> cfblk9/1(cfblk1), cfblk9/3(cfblk14), cfblk14/1, cfblk15/1, cfblk16/1
  cfblk9/3(cfblk16) -> cfblk4/1, cfblk13/1
  cfblk7/2(cfblk7) -> cfblk9/2(cfblk13)
  cfblk9/1(cfblk2) -> cfblk11/1
  cfblk11/1 -> cfblk6/2(cfblk17)
  cfblk9/2(cfblk15) -> cfblk12/1
  cfblk12/1 -> cfblk8/2(cfblk10)
  cfblk13/1 -> cfblk7/3(cfblk5)
  cfblk14/1 -> cfblk7/4(cfblk6)
  cfblk15/1 -> cfblk5/4(cfblk11)
  cfblk16/1 -> cfblk5/5(cfblk12)

== system model1_副本/cfblk73 ==
  cfblk1 : Inport
  cfblk9 : Inport  Port=2
  cfblk10 : Inport  Port=3
  cfblk3 : DiscreteStateSpace
  cfblk4 : simulink/Discrete/Transfer Fcn First Order  PoleZ=0.95  ICPrevOutput=0.0  DoSatur=off
  cfblk5 : Bias  Bias=[-817961956.565615]  SaturateOnIntegerOverflow=off
  cfblk6 : Constant  Value=[-384800716.714247]  SampleTime=1
  cfblk7 : Constant  Value=[286566385.221249]  SampleTime=1
  cfblk8 : Constant  Value=[191044421.069817]  SampleTime=1
  cfblk2 : Outport
  cfblk11 : Outport  Port=2
  wires:
  cfblk8/1 -> cfblk4/1
  cfblk3/1 -> cfblk2/1
  cfblk10/1 -> cfblk3/1
  cfblk9/1 -> cfblk11/1
  cfblk1/1 -> cfblk5/1

== system model1_副本/cfblk74 ==
  cfblk1 : Inport
  cfblk11 : Inport  Port=2
  cfblk12 : Inport  Port=3
  cfblk10 : Subsystem
  cfblk14 : Delay  SampleTime=1
  cfblk3 : DiscreteZeroPole  Poles=[0 0.5]  Gain=1
  cfblk4 : DiscreteFir  SampleTime=1
  cfblk5 : Sin  TimeSource=Use external signal  SampleTime=0
  cfblk6 : Sin  TimeSource=Use external signal  SampleTime=0
  cfblk7 : PermuteDimensions
  cfblk8 : Subsystem
  cfblk9 : Subsystem
  cfblk2 : Outport
  cfblk13 : Outport  Port=2
  wires:
  cfblk5/1 -> cfblk4/1, cfblk10/3(cfblk7)
  cfblk11/1 -> cfblk6/1
  cfblk9/1(cfblk2) -> cfblk2/1
  cfblk4/1 -> cfblk9/1(cfblk1)
  cfblk1/1 -> cfblk5/1
  cfblk9/2(cfblk15) -> cfblk7/1
  cfblk8/1(cfblk2) -> cfblk9/2(cfblk14)
  cfblk6/1 -> cfblk10/1(cfblk1)
  cfblk12/1 -> cfblk8/1(cfblk1)
  cfblk10/1(cfblk2) -> cfblk3/1
  cfblk7/1 -> cfblk13/1
  cfblk3/1 -> cfblk8/2(cfblk7)
  cfblk8/2(cfblk8) -> cfblk14/1
  cfblk14/1 -> cfblk10/2(cfblk6)

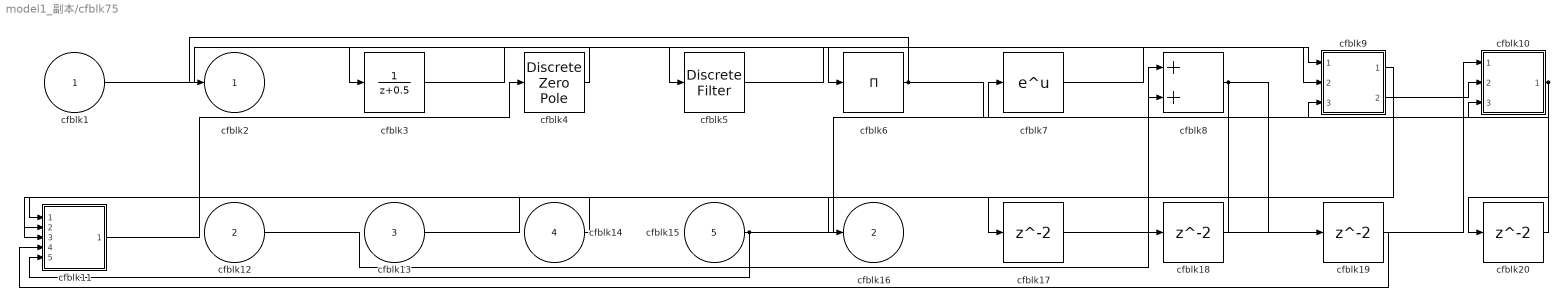
== system model1_副本/cfblk75 ==
  cfblk1 : Inport
  cfblk12 : Inport  Port=2
  cfblk13 : Inport  Port=3
  cfblk14 : Inport  Port=4
  cfblk15 : Inport  Port=5
  cfblk10 : Subsystem
  cfblk11 : Subsystem
  cfblk{17..20} (4 alike) : Delay  SampleTime=1
  cfblk3 : DiscreteTransferFcn  SampleTime=1
  cfblk4 : DiscreteZeroPole  Poles=[0 0.5]  Gain=1
  cfblk5 : DiscreteFilter  SampleTime=1
  cfblk6 : Product  Inputs=*
  cfblk7 : Math
  cfblk8 : Sum
  cfblk9 : Subsystem
  cfblk2 : Outport
  cfblk16 : Outport  Port=2
  wires:
  cfblk11/1(cfblk2) -> cfblk4/1
  cfblk15/1 -> cfblk7/1, cfblk11/5(cfblk12)
  cfblk4/1 -> cfblk3/1
  cfblk13/1 -> cfblk16/1
  cfblk3/1 -> cfblk6/1
  cfblk1/1 -> cfblk5/1
  cfblk12/1 -> cfblk8/1
  cfblk6/1 -> cfblk2/1, cfblk10/3(cfblk11)
  cfblk10/1(cfblk2) -> cfblk8/2, cfblk20/1
  cfblk14/1 -> cfblk11/1(cfblk1)
  cfblk8/1 -> cfblk17/1, cfblk18/1, cfblk19/1
  cfblk5/1 -> cfblk9/1(cfblk1)
  cfblk7/1 -> cfblk9/2(cfblk8)
  cfblk9/1(cfblk2) -> cfblk11/2(cfblk9)
  cfblk9/2(cfblk10) -> cfblk10/2(cfblk10)
  cfblk17/1 -> cfblk10/1(cfblk1)
  cfblk18/1 -> cfblk11/3(cfblk10)
  cfblk19/1 -> cfblk11/4(cfblk11)
  cfblk20/1 -> cfblk9/3(cfblk9)

== system model1_副本/cfblk76 ==
  cfblk1 : Inport
  cfblk10 : Inport  Port=2
  cfblk11 : Inport  Port=3
  cfblk12 : Delay  SampleTime=1
  cfblk3 : Sum  Inputs=+
  cfblk4 : Product
  cfblk5 : Constant  Value=[-80085410.240135]  SampleTime=1
  cfblk6 : Constant  Value=[851334714.149209]  SampleTime=1
  cfblk7 : Subsystem
  cfblk8 : Subsystem
  cfblk9 : Subsystem
  cfblk2 : Outport
  wires:
  cfblk8/1(cfblk2) -> cfblk9/1(cfblk1)
  cfblk7/1(cfblk2) -> cfblk2/1
  cfblk1/1 -> cfblk8/2(cfblk6)
  cfblk10/1 -> cfblk8/3(cfblk7)
  cfblk9/2(cfblk7) -> cfblk3/1
  cfblk6/1 -> cfblk4/1, cfblk7/5(cfblk14)
  cfblk11/1 -> cfblk4/2
  cfblk9/3(cfblk8) -> cfblk7/1(cfblk1)
  cfblk3/1 -> cfblk7/2(cfblk11)
  cfblk5/1 -> cfblk7/3(cfblk12)
  cfblk4/1 -> cfblk7/4(cfblk13)
  cfblk9/1(cfblk2) -> cfblk12/1
  cfblk12/1 -> cfblk8/1(cfblk1)

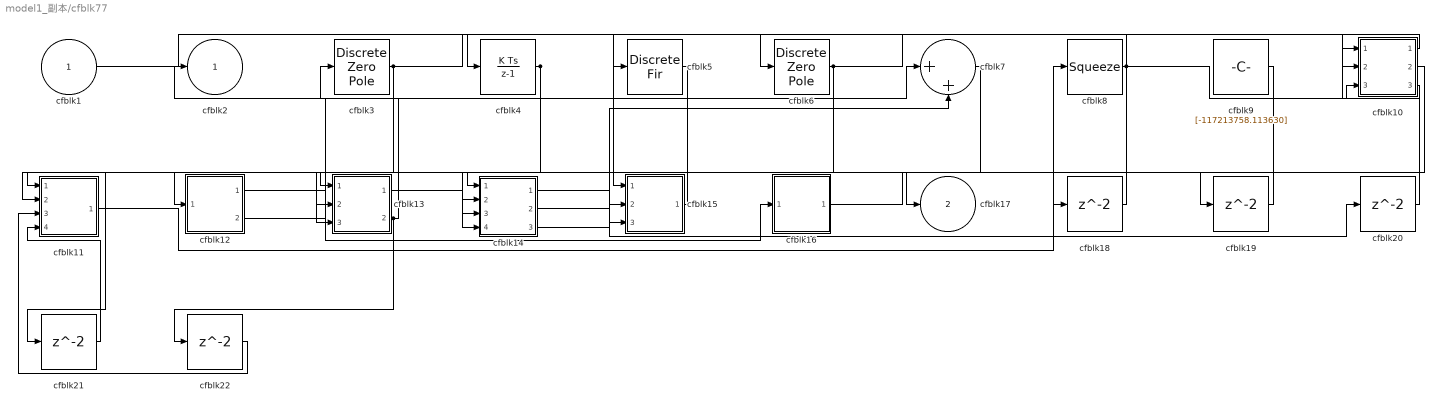
== system model1_副本/cfblk77 ==
  cfblk1 : Inport
  cfblk10 : Subsystem
  cfblk11 : Subsystem
  cfblk12 : Subsystem
  cfblk13 : Subsystem
  cfblk14 : Subsystem
  cfblk15 : Subsystem
  cfblk16 : Subsystem
  cfblk{18..22} (5 alike) : Delay  SampleTime=1
  cfblk3 : DiscreteZeroPole  Poles=[0 0.5]  Gain=1
  cfblk4 : DiscreteIntegrator  ICPrevOutput=DiscIntNeverNeededParam  ICPrevScaledInput=DiscIntNeverNeededParam
  cfblk5 : DiscreteFir  SampleTime=1
  cfblk6 : DiscreteZeroPole  Poles=[0 0.5]  Gain=1
  cfblk7 : Sum  Inputs=|++
  cfblk8 : Squeeze
  cfblk9 : Constant  Value=[-117213758.113630]  SampleTime=1
  cfblk2 : Outport
  cfblk17 : Outport  Port=2
  wires:
  cfblk12/1(cfblk2) -> cfblk16/1(cfblk1)
  cfblk11/1(cfblk2) -> cfblk8/1
  cfblk10/1(cfblk2) -> cfblk15/1(cfblk1)
  cfblk6/1 -> cfblk12/1(cfblk1), cfblk10/2(cfblk9)
  cfblk5/1 -> cfblk11/2(cfblk15)
  cfblk12/2(cfblk8) -> cfblk7/1
  cfblk9/1 -> cfblk15/2(cfblk13)
  cfblk1/1 -> cfblk5/1
  cfblk7/1 -> cfblk17/1
  cfblk10/2(cfblk11) -> cfblk14/1(cfblk1)
  cfblk8/1 -> cfblk4/1, cfblk14/4(cfblk13), cfblk13/3(cfblk7), cfblk10/3(cfblk10)
  cfblk13/1(cfblk2) -> cfblk15/3(cfblk14)
  cfblk13/2(cfblk8) -> cfblk3/1, cfblk22/1
  cfblk10/3(cfblk12) -> cfblk14/2(cfblk11)
  cfblk3/1 -> cfblk6/1, cfblk21/1
  cfblk15/1(cfblk2) -> cfblk2/1
  cfblk14/3(cfblk15) -> cfblk7/2
  cfblk4/1 -> cfblk13/2(cfblk6), cfblk14/3(cfblk12)
  cfblk16/1(cfblk2) -> cfblk18/1
  cfblk18/1 -> cfblk13/1(cfblk1)
  cfblk14/1(cfblk2) -> cfblk19/1
  cfblk19/1 -> cfblk11/1(cfblk1)
  cfblk14/2(cfblk14) -> cfblk20/1
  cfblk20/1 -> cfblk10/1(cfblk1)
  cfblk21/1 -> cfblk11/4(cfblk17)
  cfblk22/1 -> cfblk11/3(cfblk16)

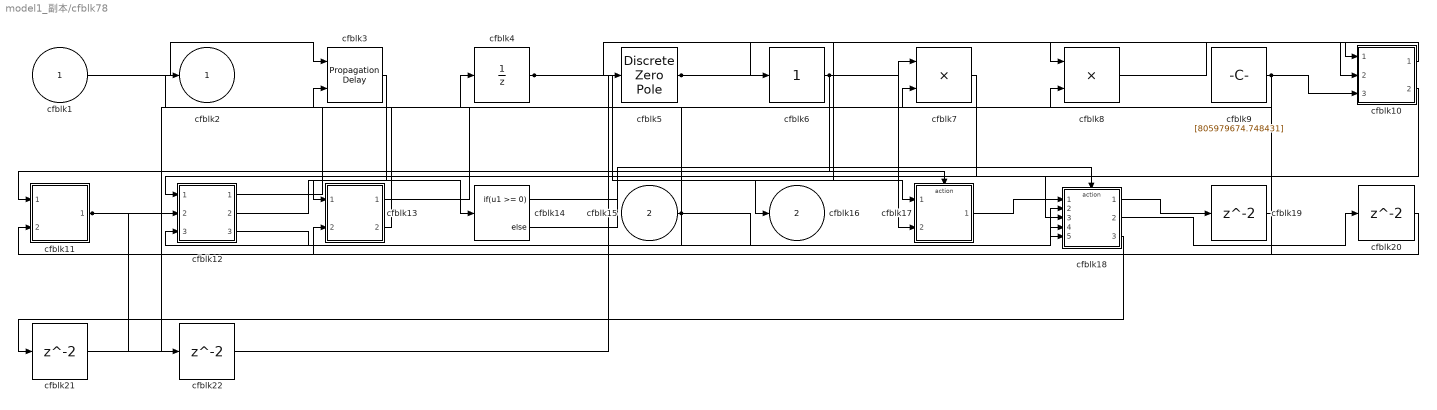
== system model1_副本/cfblk78 ==
  cfblk1 : Inport
  cfblk15 : Inport  Port=2
  cfblk10 : Subsystem
  cfblk11 : Subsystem
  cfblk12 : Subsystem
  cfblk13 : Subsystem
  cfblk14 : If  IfExpression=u1 >= 0  SampleTime=1
  cfblk17 : Subsystem  TreatAsAtomicUnit=on
  cfblk18 : Subsystem  TreatAsAtomicUnit=on
  cfblk{19..22} (4 alike) : Delay  SampleTime=1
  cfblk3 : PropagationDelay  SampleTime=1
  cfblk4 : UnitDelay  HasFrameUpgradeWarning=on
  cfblk5 : DiscreteZeroPole  Poles=[0 0.5]  Gain=1
  cfblk6 : simulink/Math Operations/Slider Gain  gain=1  low=0  high=2
  cfblk7 : Product  Inputs=**
  cfblk8 : Product
  cfblk9 : Constant  Value=[805979674.748431]  SampleTime=1
  cfblk2 : Outport
  cfblk16 : Outport  Port=2
  wires:
  cfblk5/1 -> cfblk6/1, cfblk8/1
  cfblk17/1(cfblk2) -> cfblk18/1(cfblk1)
  cfblk10/1(cfblk2) -> cfblk16/1
  cfblk6/1 -> cfblk11/1(cfblk1), cfblk18/3(cfblk13)
  cfblk4/1 -> cfblk17/1(cfblk1), cfblk10/2(cfblk9)
  cfblk13/1(cfblk2) -> cfblk7/2
  cfblk11/1(cfblk2) -> cfblk8/2, cfblk22/1
  cfblk9/1 -> cfblk11/2(cfblk9), cfblk10/3(cfblk10)
  cfblk12/1(cfblk2) -> cfblk4/1
  cfblk1/1 -> cfblk3/1
  cfblk15/1 -> cfblk3/2, cfblk18/4(cfblk14), cfblk12/3(cfblk12), cfblk18/5(cfblk15)
  cfblk3/1 -> cfblk13/1(cfblk1)
  cfblk8/1 -> cfblk10/1(cfblk1)
  cfblk12/2(cfblk13) -> cfblk14/1
  cfblk13/2(cfblk13) -> cfblk2/1
  cfblk7/1 -> cfblk12/1(cfblk1)
  cfblk10/2(cfblk11) -> cfblk17/2(cfblk7)
  cfblk12/3(cfblk14) -> cfblk18/2(cfblk12)
  cfblk14/1 -> cfblk17/Action
  cfblk14/2 -> cfblk18/Action
  cfblk18/1(cfblk2) -> cfblk19/1
  cfblk19/1 -> cfblk7/1
  cfblk18/2(cfblk16) -> cfblk20/1
  cfblk20/1 -> cfblk13/2(cfblk12)
  cfblk18/3(cfblk17) -> cfblk21/1
  cfblk21/1 -> cfblk12/2(cfblk11)
  cfblk22/1 -> cfblk5/1
